simulink model "chap3_2sim"  (R2022a)
settings: Solver=VariableStepAuto  StartTime=0.0  StopTime=40  RelTol=1e-3
settings Model: Creator=Administrator  LastModifiedBy=Administrator

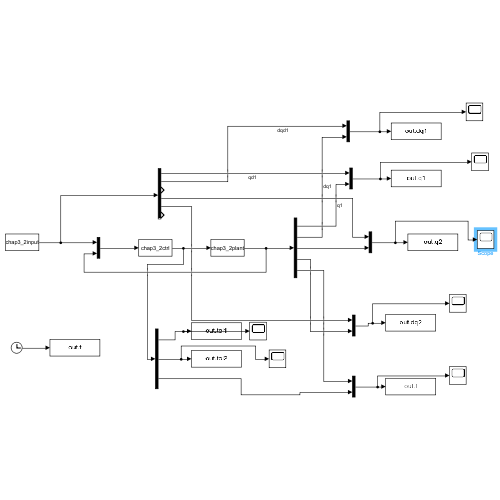
[thumbnail: Simulink's stored preview of the top-level diagram]
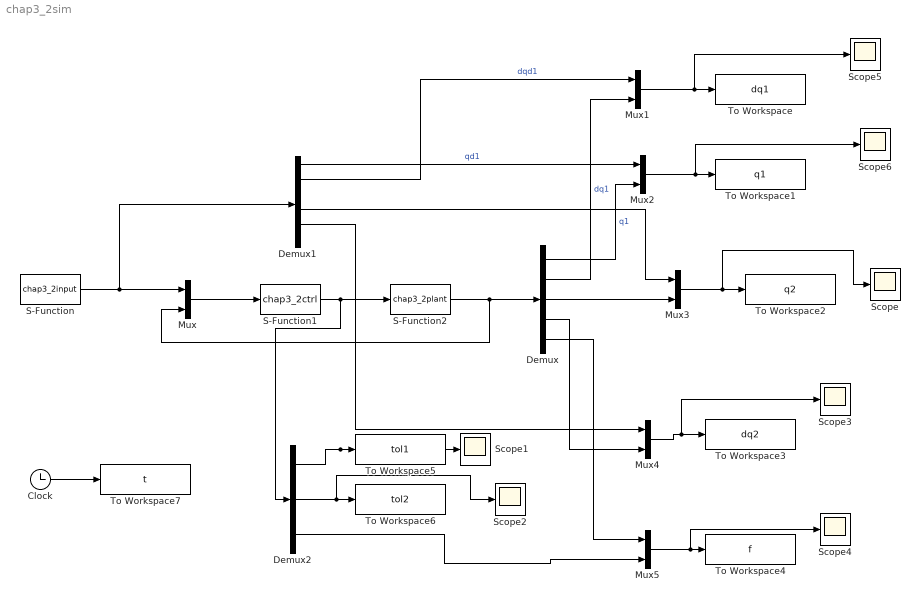
== system chap3_2sim ==
  Clock : Clock
  Demux : Demux  Outputs=5
  Demux1 : Demux  Outputs=6
  Demux2 : Demux  Outputs=3
  Mux{,1..5} (6 alike) : Mux  Inputs=2
  S-Function : S-Function  FunctionName=chap3_2input  SFunctionDeploymentMode=off  EnableBusSupport=off
  S-Function1 : S-Function  FunctionName=chap3_2ctrl  SFunctionDeploymentMode=off  EnableBusSupport=off
  S-Function2 : S-Function  FunctionName=chap3_2plant  SFunctionDeploymentMode=off  EnableBusSupport=off
  Scope{,1..6} (7 alike) : Scope
  To Workspace : ToWorkspace  VariableName=dq1  SaveFormat=Timeseries  SampleTime=-1
  To Workspace1 : ToWorkspace  VariableName=q1  SaveFormat=Timeseries  SampleTime=-1
  To Workspace2 : ToWorkspace  VariableName=q2  SaveFormat=Timeseries  SampleTime=-1
  To Workspace3 : ToWorkspace  VariableName=dq2  SaveFormat=Timeseries  SampleTime=-1
  To Workspace4 : ToWorkspace  VariableName=f  SaveFormat=Timeseries  SampleTime=-1
  To Workspace5 : ToWorkspace  VariableName=tol1  SaveFormat=Timeseries  SampleTime=-1
  To Workspace6 : ToWorkspace  VariableName=tol2  SaveFormat=Timeseries  SampleTime=-1
  To Workspace7 : ToWorkspace  VariableName=t  SaveFormat=Timeseries  SampleTime=-1
  wires:
  S-Function/1 -> Demux1/1, Mux/1
  Mux/1 -> S-Function1/1
  S-Function1/1 -> Demux2/1, S-Function2/1
  S-Function2/1 -> Mux/2, Demux/1
  Demux1/1 -> Mux2/1  "qd1"
  Demux1/2 -> Mux1/1  "dqd1"
  Demux/2 -> Mux1/2  "dq1"
  Mux1/1 -> Scope5/1, To Workspace/1
  Demux/1 -> Mux2/2  "q1"
  Mux2/1 -> Scope6/1, To Workspace1/1
  Clock/1 -> To Workspace7/1
  Demux/5 -> Mux5/1
  Demux/3 -> Mux3/2
  Mux3/1 -> Scope/1, To Workspace2/1
  Demux/4 -> Mux4/2
  Demux1/4 -> Mux3/1
  Demux1/5 -> Mux4/1
  Mux4/1 -> Scope3/1, To Workspace3/1
  Demux2/1 -> Scope1/1, To Workspace5/1
  Demux2/2 -> Scope2/1, To Workspace6/1
  Demux2/3 -> Mux5/2
  Mux5/1 -> Scope4/1, To Workspace4/1
